simulink model "PlatoonWithLateralControlExample"  (R2021b)
settings: Solver=FixedStepAuto  StartTime=0  StopTime=180  RelTol=1e-3
values from neighbouring files (symbols this model uses):
  C = [1 0 0 0; 0 1 0 0]    [truck_trailer_model.m]
undefined symbols (not defined in the file or in its folder): amp, follow1_pose0, follow2_pose0, follow3_pose0, front_pose0, lead_pose0, Ts, Vx0
libraries: drivingscenarioandsensors x5, sim3dautolib x5, sim3dlib x1
settings Model: PauseTimes=200  Creator=gabep  LastModifiedBy=gabep
settings DataIOCC: SaveFormat=Array  ReturnWorkspaceOutputs=off
settings OptimizationCC: BlockReduction=off  BufferReuse=off
settings DebuggingCC: AlgebraicLoopMsg=none  UnconnectedInputMsg=none  UnconnectedOutputMsg=none  UnconnectedLineMsg=none

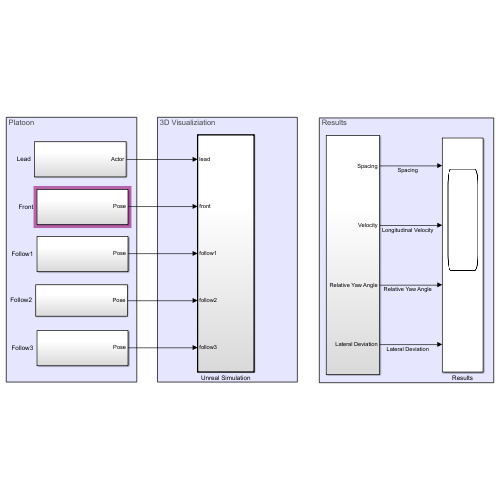
[thumbnail: Simulink's stored preview of the top-level diagram]
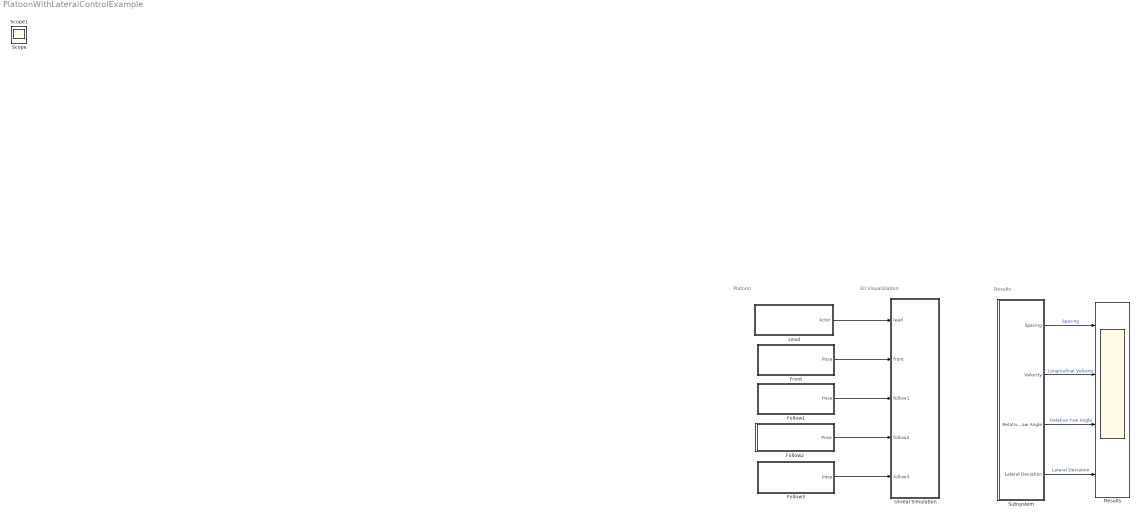
== system PlatoonWithLateralControlExample ==
  note: Results
  note: Platoon
  note: 3D Visualiziation
  Follow1 : Subsystem
      settings: PortSchema="{\"entries\":[{\"content\":{\"sides\":[{\"content\":{\"connectorIds\":[]},\"type\":\"ConnectorPlacement.EquallySpacedRectSide\",\"uuid\":\"e54d76f8-8c49-4840-b6a9-58e08104dcc1\"},{\"content\":{\"connectorIds\":[],\"side\":\"RIGHT\"},\"type\":\"ConnectorPlacement.EquallySpacedRectSide\",\"uuid\":\"16d97aed-590d-4da6-9d09-35159b7cd9d4\"},{\"content\":{\"connectorIds\":[\"Out1\"],\"side\":\"TOP\"},\"type\":\"ConnectorPlacement.EquallySpacedRectSide\",\"uuid\":\"c2bfedc8-00ba-418d-b164-6614631c3f94\"}]},\"type\":\"ConnectorPlacement.EquallySpacedConnector\",\"uuid\":\"51c3c2ba-a1bc-4371-a1ec-9944d72910ba\"}],\"packageUris\":[\"http://schema.mathworks.com/mf0/Connector/R2020b\"],\"version\":\"1.0\"}"
  Follow2 : Subsystem
      settings: PortSchema="{\"entries\":[{\"content\":{\"sides\":[{\"content\":{\"connectorIds\":[]},\"type\":\"ConnectorPlacement.EquallySpacedRectSide\",\"uuid\":\"06893071-ec21-4ffc-a054-06bfa92a0eac\"},{\"content\":{\"connectorIds\":[],\"side\":\"RIGHT\"},\"type\":\"ConnectorPlacement.EquallySpacedRectSide\",\"uuid\":\"1cbc90e1-f519-4952-8f8a-3c170042a637\"},{\"content\":{\"connectorIds\":[\"Out1\"],\"side\":\"TOP\"},\"type\":\"ConnectorPlacement.EquallySpacedRectSide\",\"uuid\":\"b6adb661-09de-4d57-bc58-bfba7e0f462d\"}]},\"type\":\"ConnectorPlacement.EquallySpacedConnector\",\"uuid\":\"b02e6905-9b80-44f2-a3ff-3310e2960530\"}],\"packageUris\":[\"http://schema.mathworks.com/mf0/Connector/R2020b\"],\"version\":\"1.0\"}"
  Follow3 : Subsystem
      settings: PortSchema="{\"entries\":[{\"content\":{\"sides\":[{\"content\":{\"connectorIds\":[]},\"type\":\"ConnectorPlacement.EquallySpacedRectSide\",\"uuid\":\"e54d76f8-8c49-4840-b6a9-58e08104dcc1\"},{\"content\":{\"connectorIds\":[],\"side\":\"RIGHT\"},\"type\":\"ConnectorPlacement.EquallySpacedRectSide\",\"uuid\":\"16d97aed-590d-4da6-9d09-35159b7cd9d4\"},{\"content\":{\"connectorIds\":[\"Out1\"],\"side\":\"TOP\"},\"type\":\"ConnectorPlacement.EquallySpacedRectSide\",\"uuid\":\"c2bfedc8-00ba-418d-b164-6614631c3f94\"}]},\"type\":\"ConnectorPlacement.EquallySpacedConnector\",\"uuid\":\"51c3c2ba-a1bc-4371-a1ec-9944d72910ba\"}],\"packageUris\":[\"http://schema.mathworks.com/mf0/Connector/R2020b\"],\"version\":\"1.0\"}"
  Front : Subsystem
      settings: PortSchema="{\"entries\":[{\"content\":{\"sides\":[{\"content\":{\"connectorIds\":[]},\"type\":\"ConnectorPlacement.EquallySpacedRectSide\",\"uuid\":\"e54d76f8-8c49-4840-b6a9-58e08104dcc1\"},{\"content\":{\"connectorIds\":[],\"side\":\"RIGHT\"},\"type\":\"ConnectorPlacement.EquallySpacedRectSide\",\"uuid\":\"16d97aed-590d-4da6-9d09-35159b7cd9d4\"},{\"content\":{\"connectorIds\":[\"Out1\"],\"side\":\"TOP\"},\"type\":\"ConnectorPlacement.EquallySpacedRectSide\",\"uuid\":\"c2bfedc8-00ba-418d-b164-6614631c3f94\"}]},\"type\":\"ConnectorPlacement.EquallySpacedConnector\",\"uuid\":\"51c3c2ba-a1bc-4371-a1ec-9944d72910ba\"}],\"packageUris\":[\"http://schema.mathworks.com/mf0/Connector/R2020b\"],\"version\":\"1.0\"}"
  Lead : Subsystem
      settings: PortSchema="{\"entries\":[{\"content\":{\"sides\":[{\"content\":{\"connectorIds\":[]},\"type\":\"ConnectorPlacement.EquallySpacedRectSide\",\"uuid\":\"e54d76f8-8c49-4840-b6a9-58e08104dcc1\"},{\"content\":{\"connectorIds\":[],\"side\":\"RIGHT\"},\"type\":\"ConnectorPlacement.EquallySpacedRectSide\",\"uuid\":\"16d97aed-590d-4da6-9d09-35159b7cd9d4\"},{\"content\":{\"connectorIds\":[\"Out1\"],\"side\":\"TOP\"},\"type\":\"ConnectorPlacement.EquallySpacedRectSide\",\"uuid\":\"c2bfedc8-00ba-418d-b164-6614631c3f94\"}]},\"type\":\"ConnectorPlacement.EquallySpacedConnector\",\"uuid\":\"51c3c2ba-a1bc-4371-a1ec-9944d72910ba\"}],\"packageUris\":[\"http://schema.mathworks.com/mf0/Connector/R2020b\"],\"version\":\"1.0\"}"
  Results : Scope  NumInputPorts=4
  Subsystem : Subsystem
  Unreal Simulation : Subsystem  TreatAsAtomicUnit=on
  Scope : Scope
  Scope1 : Scope
  wires:
  Lead/1(Actor) -> Unreal Simulation/1(lead)
  Front/1(Pose) -> Unreal Simulation/2(front)
  Follow1/1(Pose) -> Unreal Simulation/3(follow1)
  Follow2/1(Pose) -> Unreal Simulation/4(follow2)
  Follow3/1(Pose) -> Unreal Simulation/5(follow3)
  Subsystem/1(Spacing) -> Results/1  "Spacing"
  Subsystem/2(Velocity) -> Results/2  "Longitudinal Velocity"
  Subsystem/4(Lateral Deviation) -> Results/4  "Lateral Deviation"
  Subsystem/3(Relative Yaw Angle) -> Results/3  "Relative Yaw Angle"

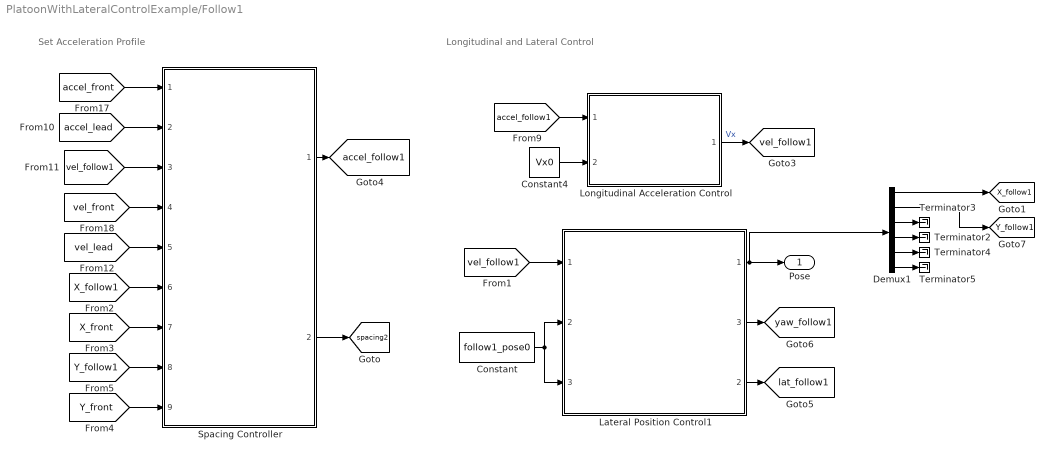
== system PlatoonWithLateralControlExample/Follow1 ==
  note: Set Acceleration Profile
  note: Longitudinal and Lateral Control
  Constant : Constant  Value=follow1_pose0
  Constant4 : Constant  Value=Vx0
  Demux1 : Demux  Outputs=6
  Lateral Position Control1 : Subsystem  ReferencedSubsystem=Lateral_Position_Control
      settings: PortSchema="{\"entries\":[{\"content\":{\"sides\":[{\"content\":{\"connectorIds\":[\"In1\",\"In2\",\"In3\"]},\"type\":\"ConnectorPlacement.EquallySpacedRectSide\",\"uuid\":\"be29c3cb-f330-4838-b745-538466c19ec8\"},{\"content\":{\"connectorIds\":[\"Out1\",\"Out3\",\"Out2\"],\"side\":\"RIGHT\"},\"type\":\"ConnectorPlacement.EquallySpacedRectSide\",\"uuid\":\"f85912df-f35d-4388-8854-cabd9b7a9775\"},{\"content\":{\"connectorIds\":[],\"side\":\"TOP\"},\"type\":\"ConnectorPlacement.EquallySpacedRectSide\",\"uuid\":\"58ed6a5b-2636-4a09-8dd1-9e23de881849\"}]},\"type\":\"ConnectorPlacement.EquallySpacedConnector\",\"uuid\":\"159292d7-4540-43fd-9ff3-bfddba653fcb\"}],\"packageUris\":[\"http://schema.mathworks.com/mf0/Connector/R2020b\"],\"version\":\"1.0\"}"
  Longitudinal Acceleration Control : Subsystem  ReferencedSubsystem=Longitudinal_Acceleration_Control
  Spacing Controller : Subsystem  ReferencedSubsystem=spacing_controller
  Terminator{2..5} (4 alike) : Terminator
  Pose : Outport
  tag scope: X_follow1=global, Y_follow1=global, accel_follow1=global, lat_follow1=global, spacing2=global, vel_follow1=global, yaw_follow1=global
  wires:
  Constant4/1 -> Longitudinal Acceleration Control/2
  [accel_follow1] -> Longitudinal Acceleration Control/1
  Longitudinal Acceleration Control/1 -> [vel_follow1]  "Vx"
  Lateral Position Control1/3 -> [yaw_follow1]
  Lateral Position Control1/2 -> [lat_follow1]
  [vel_follow1] -> Lateral Position Control1/1
  Constant/1 -> Lateral Position Control1/3, Lateral Position Control1/2
  Spacing Controller/2 -> [spacing2]
  [accel_front] -> Spacing Controller/1
  [accel_lead] -> Spacing Controller/2
  [vel_follow1] -> Spacing Controller/3
  [vel_front] -> Spacing Controller/4
  [vel_lead] -> Spacing Controller/5
  Spacing Controller/1 -> [accel_follow1]
  [X_front] -> Spacing Controller/7
  [X_follow1] -> Spacing Controller/6
  Demux1/4 -> Terminator2/1
  Demux1/6 -> Terminator5/1
  Demux1/2 -> [Y_follow1]
  Demux1/1 -> [X_follow1]
  Demux1/5 -> Terminator4/1
  Demux1/3 -> Terminator3/1
  Lateral Position Control1/1 -> Demux1/1, Pose/1
  [Y_front] -> Spacing Controller/9
  [Y_follow1] -> Spacing Controller/8

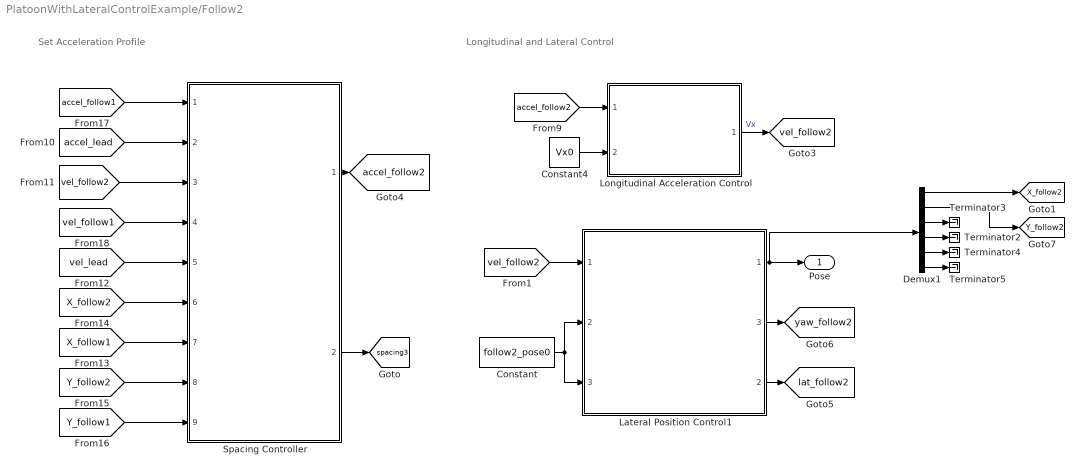
== system PlatoonWithLateralControlExample/Follow2 ==
  note: Set Acceleration Profile
  note: Longitudinal and Lateral Control
  Constant : Constant  Value=follow2_pose0
  Constant4 : Constant  Value=Vx0
  Demux1 : Demux  Outputs=6
  Lateral Position Control1 : Subsystem  ReferencedSubsystem=Lateral_Position_Control
      settings: PortSchema="{\"entries\":[{\"content\":{\"sides\":[{\"content\":{\"connectorIds\":[\"In1\",\"In2\",\"In3\"]},\"type\":\"ConnectorPlacement.EquallySpacedRectSide\",\"uuid\":\"be29c3cb-f330-4838-b745-538466c19ec8\"},{\"content\":{\"connectorIds\":[\"Out1\",\"Out3\",\"Out2\"],\"side\":\"RIGHT\"},\"type\":\"ConnectorPlacement.EquallySpacedRectSide\",\"uuid\":\"f85912df-f35d-4388-8854-cabd9b7a9775\"},{\"content\":{\"connectorIds\":[],\"side\":\"TOP\"},\"type\":\"ConnectorPlacement.EquallySpacedRectSide\",\"uuid\":\"58ed6a5b-2636-4a09-8dd1-9e23de881849\"}]},\"type\":\"ConnectorPlacement.EquallySpacedConnector\",\"uuid\":\"159292d7-4540-43fd-9ff3-bfddba653fcb\"}],\"packageUris\":[\"http://schema.mathworks.com/mf0/Connector/R2020b\"],\"version\":\"1.0\"}"
  Longitudinal Acceleration Control : Subsystem  ReferencedSubsystem=Longitudinal_Acceleration_Control
  Spacing Controller : Subsystem  ReferencedSubsystem=spacing_controller
  Terminator{2..5} (4 alike) : Terminator
  Pose : Outport
  tag scope: X_follow2=global, Y_follow2=global, accel_follow2=global, lat_follow2=global, spacing3=global, vel_follow2=global, yaw_follow2=global
  wires:
  Constant4/1 -> Longitudinal Acceleration Control/2
  [accel_follow2] -> Longitudinal Acceleration Control/1
  Longitudinal Acceleration Control/1 -> [vel_follow2]  "Vx"
  [Y_follow2] -> Spacing Controller/8
  [X_follow1] -> Spacing Controller/7
  Spacing Controller/1 -> [accel_follow2]
  [vel_follow2] -> Spacing Controller/3
  [vel_lead] -> Spacing Controller/5
  [accel_lead] -> Spacing Controller/2
  [Y_follow1] -> Spacing Controller/9
  [X_follow2] -> Spacing Controller/6
  [accel_follow1] -> Spacing Controller/1
  [vel_follow1] -> Spacing Controller/4
  Spacing Controller/2 -> [spacing3]
  Lateral Position Control1/3 -> [yaw_follow2]
  Lateral Position Control1/2 -> [lat_follow2]
  [vel_follow2] -> Lateral Position Control1/1
  Constant/1 -> Lateral Position Control1/3, Lateral Position Control1/2
  Demux1/3 -> Terminator3/1
  Demux1/5 -> Terminator4/1
  Demux1/1 -> [X_follow2]
  Demux1/6 -> Terminator5/1
  Demux1/2 -> [Y_follow2]
  Demux1/4 -> Terminator2/1
  Lateral Position Control1/1 -> Demux1/1, Pose/1

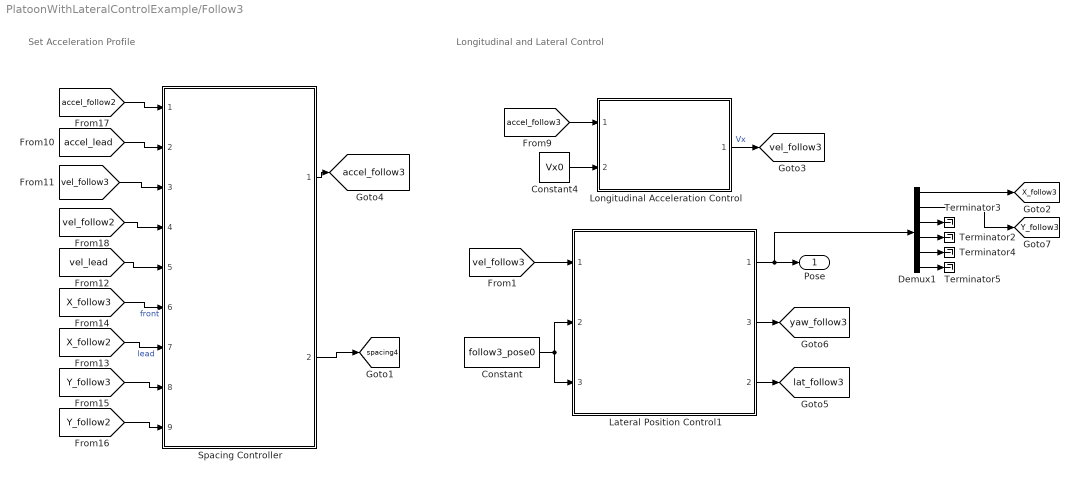
== system PlatoonWithLateralControlExample/Follow3 ==
  note: Set Acceleration Profile
  note: Longitudinal and Lateral Control
  Constant : Constant  Value=follow3_pose0
  Constant4 : Constant  Value=Vx0
  Demux1 : Demux  Outputs=6
  Lateral Position Control1 : Subsystem  ReferencedSubsystem=Lateral_Position_Control
      settings: PortSchema="{\"entries\":[{\"content\":{\"sides\":[{\"content\":{\"connectorIds\":[\"In1\",\"In2\",\"In3\"]},\"type\":\"ConnectorPlacement.EquallySpacedRectSide\",\"uuid\":\"be29c3cb-f330-4838-b745-538466c19ec8\"},{\"content\":{\"connectorIds\":[\"Out1\",\"Out3\",\"Out2\"],\"side\":\"RIGHT\"},\"type\":\"ConnectorPlacement.EquallySpacedRectSide\",\"uuid\":\"f85912df-f35d-4388-8854-cabd9b7a9775\"},{\"content\":{\"connectorIds\":[],\"side\":\"TOP\"},\"type\":\"ConnectorPlacement.EquallySpacedRectSide\",\"uuid\":\"58ed6a5b-2636-4a09-8dd1-9e23de881849\"}]},\"type\":\"ConnectorPlacement.EquallySpacedConnector\",\"uuid\":\"159292d7-4540-43fd-9ff3-bfddba653fcb\"}],\"packageUris\":[\"http://schema.mathworks.com/mf0/Connector/R2020b\"],\"version\":\"1.0\"}"
  Longitudinal Acceleration Control : Subsystem  ReferencedSubsystem=Longitudinal_Acceleration_Control
  Spacing Controller : Subsystem  ReferencedSubsystem=spacing_controller
  Terminator{2..5} (4 alike) : Terminator
  Pose : Outport
  tag scope: X_follow3=global, Y_follow3=global, accel_follow3=global, lat_follow3=global, spacing4=global, vel_follow3=global, yaw_follow3=global
  wires:
  Constant4/1 -> Longitudinal Acceleration Control/2
  [accel_follow3] -> Longitudinal Acceleration Control/1
  Longitudinal Acceleration Control/1 -> [vel_follow3]  "Vx"
  [Y_follow3] -> Spacing Controller/8
  [X_follow2] -> Spacing Controller/7  "lead"
  [vel_follow3] -> Spacing Controller/3
  [vel_lead] -> Spacing Controller/5
  [accel_lead] -> Spacing Controller/2
  [Y_follow2] -> Spacing Controller/9
  [X_follow3] -> Spacing Controller/6  "front"
  [accel_follow2] -> Spacing Controller/1
  [vel_follow2] -> Spacing Controller/4
  Spacing Controller/1 -> [accel_follow3]
  Spacing Controller/2 -> [spacing4]
  Lateral Position Control1/3 -> [yaw_follow3]
  Lateral Position Control1/2 -> [lat_follow3]
  [vel_follow3] -> Lateral Position Control1/1
  Constant/1 -> Lateral Position Control1/3, Lateral Position Control1/2
  Demux1/3 -> Terminator3/1
  Demux1/5 -> Terminator4/1
  Demux1/1 -> [X_follow3]
  Demux1/6 -> Terminator5/1
  Demux1/2 -> [Y_follow3]
  Demux1/4 -> Terminator2/1
  Lateral Position Control1/1 -> Demux1/1, Pose/1

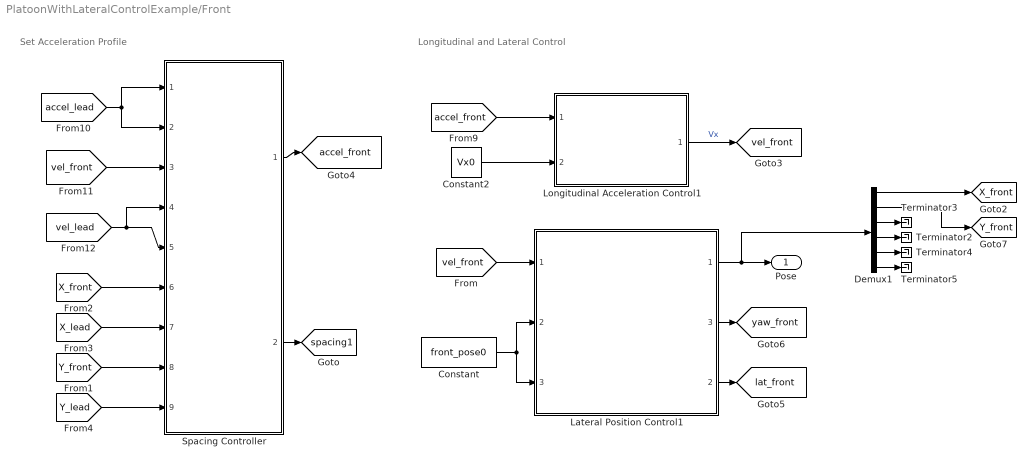
== system PlatoonWithLateralControlExample/Front ==
  note: Longitudinal and Lateral Control
  note: Set Acceleration Profile
  Constant : Constant  Value=front_pose0
  Constant2 : Constant  Value=Vx0
  Demux1 : Demux  Outputs=6
  Lateral Position Control1 : Subsystem  ReferencedSubsystem=Lateral_Position_Control
      settings: PortSchema="{\"entries\":[{\"content\":{\"sides\":[{\"content\":{\"connectorIds\":[\"In1\",\"In2\",\"In3\"]},\"type\":\"ConnectorPlacement.EquallySpacedRectSide\",\"uuid\":\"be29c3cb-f330-4838-b745-538466c19ec8\"},{\"content\":{\"connectorIds\":[\"Out1\",\"Out3\",\"Out2\"],\"side\":\"RIGHT\"},\"type\":\"ConnectorPlacement.EquallySpacedRectSide\",\"uuid\":\"f85912df-f35d-4388-8854-cabd9b7a9775\"},{\"content\":{\"connectorIds\":[],\"side\":\"TOP\"},\"type\":\"ConnectorPlacement.EquallySpacedRectSide\",\"uuid\":\"58ed6a5b-2636-4a09-8dd1-9e23de881849\"}]},\"type\":\"ConnectorPlacement.EquallySpacedConnector\",\"uuid\":\"159292d7-4540-43fd-9ff3-bfddba653fcb\"}],\"packageUris\":[\"http://schema.mathworks.com/mf0/Connector/R2020b\"],\"version\":\"1.0\"}"
  Longitudinal Acceleration Control1 : Subsystem  ReferencedSubsystem=Longitudinal_Acceleration_Control
  Spacing Controller : Subsystem  ReferencedSubsystem=spacing_controller
  Terminator{2..5} (4 alike) : Terminator
  Pose : Outport
  tag scope: X_front=global, Y_front=global, accel_front=global, lat_front=global, spacing1=global, vel_front=global, yaw_front=global
  wires:
  [accel_lead] -> Spacing Controller/2, Spacing Controller/1
  [vel_front] -> Spacing Controller/3
  [vel_lead] -> Spacing Controller/5, Spacing Controller/4
  Spacing Controller/1 -> [accel_front]
  Constant/1 -> Lateral Position Control1/3, Lateral Position Control1/2
  Constant2/1 -> Longitudinal Acceleration Control1/2
  [accel_front] -> Longitudinal Acceleration Control1/1
  Lateral Position Control1/2 -> [lat_front]
  Longitudinal Acceleration Control1/1 -> [vel_front]  "Vx"
  Lateral Position Control1/3 -> [yaw_front]
  [vel_front] -> Lateral Position Control1/1
  [X_front] -> Spacing Controller/6
  [X_lead] -> Spacing Controller/7
  Spacing Controller/2 -> [spacing1]
  Demux1/4 -> Terminator2/1
  Demux1/6 -> Terminator5/1
  Demux1/2 -> [Y_front]
  Demux1/1 -> [X_front]
  Demux1/5 -> Terminator4/1
  Demux1/3 -> Terminator3/1
  Lateral Position Control1/1 -> Pose/1, Demux1/1
  [Y_lead] -> Spacing Controller/9
  [Y_front] -> Spacing Controller/8

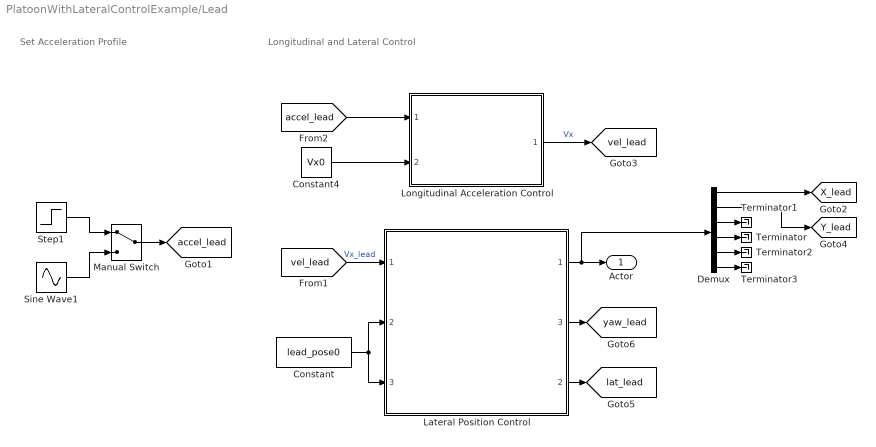
== system PlatoonWithLateralControlExample/Lead ==
  note: Set Acceleration Profile
  note: Longitudinal and Lateral Control
  Constant : Constant  Value=lead_pose0
  Constant4 : Constant  Value=Vx0
  Demux : Demux  Outputs=6
  Lateral Position Control : Subsystem  ReferencedSubsystem=Lateral_Position_Control
      settings: PortSchema="{\"entries\":[{\"content\":{\"sides\":[{\"content\":{\"connectorIds\":[\"In1\",\"In2\",\"In3\"]},\"type\":\"ConnectorPlacement.EquallySpacedRectSide\",\"uuid\":\"be29c3cb-f330-4838-b745-538466c19ec8\"},{\"content\":{\"connectorIds\":[\"Out1\",\"Out3\",\"Out2\"],\"side\":\"RIGHT\"},\"type\":\"ConnectorPlacement.EquallySpacedRectSide\",\"uuid\":\"f85912df-f35d-4388-8854-cabd9b7a9775\"},{\"content\":{\"connectorIds\":[],\"side\":\"TOP\"},\"type\":\"ConnectorPlacement.EquallySpacedRectSide\",\"uuid\":\"58ed6a5b-2636-4a09-8dd1-9e23de881849\"}]},\"type\":\"ConnectorPlacement.EquallySpacedConnector\",\"uuid\":\"159292d7-4540-43fd-9ff3-bfddba653fcb\"}],\"packageUris\":[\"http://schema.mathworks.com/mf0/Connector/R2020b\"],\"version\":\"1.0\"}"
  Longitudinal Acceleration Control : Subsystem  ReferencedSubsystem=Longitudinal_Acceleration_Control
  Manual Switch : ManualSwitch
  Sine Wave1 : Sin  Amplitude=amp  SampleTime=0
  Step1 : Step  Time=0  After=0  SampleTime=0
  Terminator{,1..3} (4 alike) : Terminator
  Actor : Outport
  tag scope: X_lead=global, Y_lead=global, accel_lead=global, lat_lead=global, vel_lead=global, yaw_lead=global
  wires:
  Constant4/1 -> Longitudinal Acceleration Control/2
  Longitudinal Acceleration Control/1 -> [vel_lead]  "Vx"
  [accel_lead] -> Longitudinal Acceleration Control/1
  Step1/1 -> Manual Switch/1
  Manual Switch/1 -> [accel_lead]
  Sine Wave1/1 -> Manual Switch/2
  Lateral Position Control/3 -> [yaw_lead]
  Lateral Position Control/2 -> [lat_lead]
  Constant/1 -> Lateral Position Control/2, Lateral Position Control/3
  [vel_lead] -> Lateral Position Control/1  "Vx_lead"
  Demux/2 -> [Y_lead]
  Lateral Position Control/1 -> Demux/1, Actor/1
  Demux/3 -> Terminator1/1
  Demux/1 -> [X_lead]
  Demux/4 -> Terminator/1
  Demux/5 -> Terminator2/1
  Demux/6 -> Terminator3/1

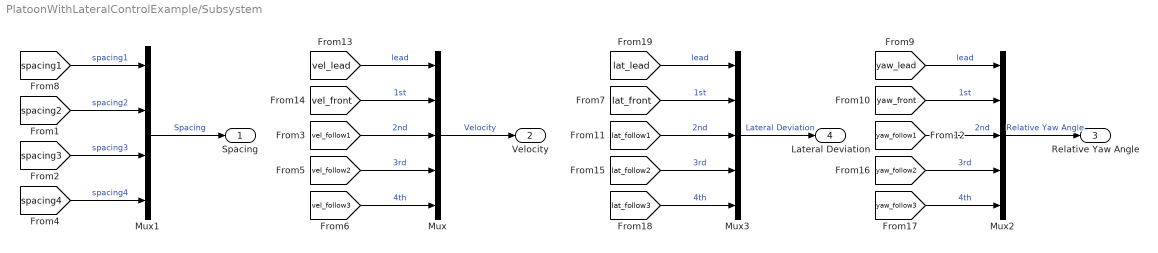
== system PlatoonWithLateralControlExample/Subsystem ==
  Mux : Mux  Inputs=5
  Mux1 : Mux
  Mux2 : Mux  Inputs=5
  Mux3 : Mux  Inputs=5
  Spacing : Outport
  Velocity : Outport  Port=2
  Relative Yaw Angle : Outport  Port=3
  Lateral Deviation : Outport  Port=4
  wires:
  [vel_follow2] -> Mux/4  "3rd"
  [vel_lead] -> Mux/1  "lead"
  [vel_front] -> Mux/2  "1st"
  [spacing3] -> Mux1/3  "spacing3"
  [vel_follow1] -> Mux/3  "2nd"
  [spacing1] -> Mux1/1  "spacing1"
  [spacing4] -> Mux1/4  "spacing4"
  [vel_follow3] -> Mux/5  "4th"
  [spacing2] -> Mux1/2  "spacing2"
  Mux/1 -> Velocity/1  "Velocity"
  Mux1/1 -> Spacing/1  "Spacing"
  Mux2/1 -> Relative Yaw Angle/1  "Relative Yaw Angle"
  [yaw_follow3] -> Mux2/5  "4th"
  [yaw_follow1] -> Mux2/3  "2nd"
  [yaw_front] -> Mux2/2  "1st"
  [yaw_follow2] -> Mux2/4  "3rd"
  [yaw_lead] -> Mux2/1  "lead"
  [lat_lead] -> Mux3/1  "lead"
  [lat_follow1] -> Mux3/3  "2nd"
  [lat_follow2] -> Mux3/4  "3rd"
  Mux3/1 -> Lateral Deviation/1  "Lateral Deviation"
  [lat_follow3] -> Mux3/5  "4th"
  [lat_front] -> Mux3/2  "1st"

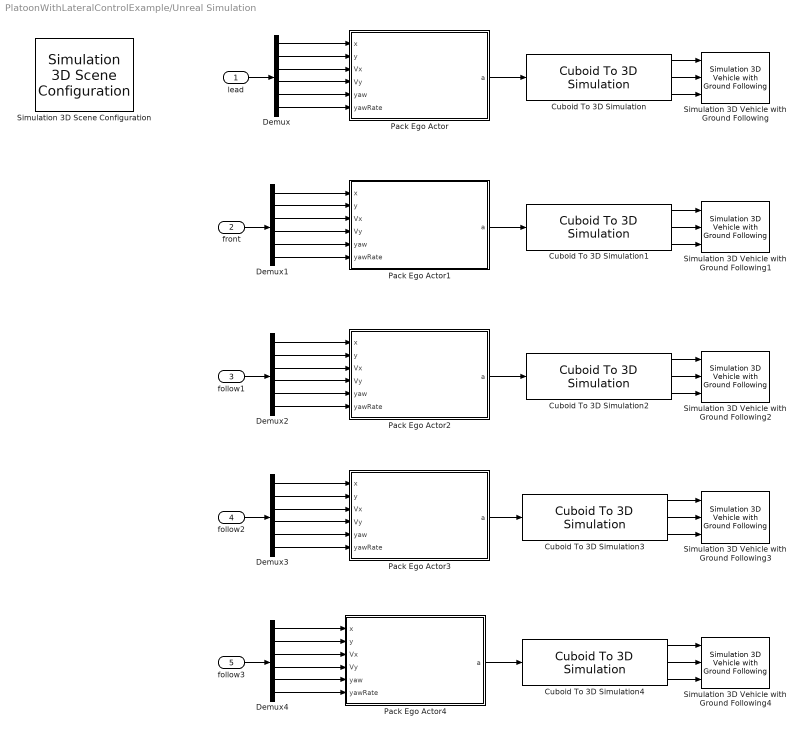
== system PlatoonWithLateralControlExample/Unreal Simulation ==
  lead : Inport
  front : Inport  Port=2
  follow1 : Inport  Port=3
  follow2 : Inport  Port=4
  follow3 : Inport  Port=5
  Cuboid To 3D Simulation{,1..4} (5 alike) : drivingscenarioandsensors/Cuboid To 3D Simulation  SpecifyActorID=off  ActorIDToConvert=1  SimulateUsing=Interpreted execution
      settings: SourceProductBaseCode=DR
  Demux{,1..4} (5 alike) : Demux  Outputs=6
  Pack Ego Actor : MATLAB Function  TreatAsAtomicUnit=on  mask{egoActorID=1}
      mask prompts: egoActorID "Ego Actor ID"
  Pack Ego Actor1 : MATLAB Function  TreatAsAtomicUnit=on  mask{egoActorID=1}
      mask prompts: egoActorID "Ego Actor ID"
  Pack Ego Actor2 : MATLAB Function  TreatAsAtomicUnit=on  mask{egoActorID=1}
      mask prompts: egoActorID "Ego Actor ID"
  Pack Ego Actor3 : MATLAB Function  TreatAsAtomicUnit=on  mask{egoActorID=1}
      mask prompts: egoActorID "Ego Actor ID"
  Pack Ego Actor4 : MATLAB Function  TreatAsAtomicUnit=on  mask{egoActorID=1}
      mask prompts: egoActorID "Ego Actor ID"
  Simulation 3D Scene Configuration : sim3dlib/Simulation 3D Scene Configuration  Priority=0  ProjectFormat_internal=Unreal Executable  ProjectFormat=Unreal Executable  SceneDesc=Curved road  ProjectName=C:\ProgramData\MATLAB\SupportPackages\R2021b\toolbox\shared\sim3dprojects\driving\RoadRunnerScenes\WindowsPackage\RRScene.exe  ScenePath=/Game/Maps/RRHighway  vehTagList={'Scene Origin';'SimulinkVehicle1';'SimulinkVehicle2';'SimulinkVehicle3';'SimulinkVehicle4';'SimulinkVehicle5'}  vehTag=SimulinkVehicle5  OpVisEn=off  Ts=Ts  EnableWindow=on  EnableWeather=off  SunAltitude=-43.200  SunAzimuth=54.0  clouds=7.0  wind=2.0  fog=0  rain=0  sensorTag=MainCamera1  sensorId=1  sensorName=MainCamera1  mountLoc=Origin  offsetFlag=off  tmountOffset=[0, 0, 0]  rmountOffset=[0, 0, 0]  HorizontalResolution=1280  VerticalResolution=720  HorizontalFOV=60  mountPoint=[0 0 0]  mountOrientation=[0 0 0]  aMode=3  ID=1
      settings: SourceProductBaseCode=AE,DR,UV,VE
      settings: AttributesFormatString=|
      | -------------------------------------
      | SceneName = %<SceneDesc>
      | Priority = %<Priority>
  Simulation 3D Vehicle with Ground Following : sim3dautolib/Simulation 3D Vehicle with Ground Following  Priority=-1  PassVehMesh=Box truck  PassVehMesh_Internal=Box truck  MeshPath=/MathWorksSimulation/Vehicles/Muscle/Meshes/SK_MuscleCar.SK_MuscleCar  TrackWidth=1.9  WheelBase=3  WheelRadius=0.35  VehColor=Blue  VehColor_Internal=Blue  InitialPos=[0,0,0]  InitialRot=[0, 0, 0]  ActorName=SimulinkVehicle1  SampleTime=-1  ActorType=SimulinkVehicle  ID=1  aMode=3  ActorTag=SimulinkVehicle1  CoordinateScheme=ISO  VehLightsControl=off  HeadlightColor=[ 1, 1, 1 ]  HighBeamIntensity=100000  LowBeamIntensity=60000  HighBeamConeAngle=70  LowBeamConeAngle=70  LeftHeadlightOrientation=[ 0, 0 ]  RightHeadlightOrientation=[ 0, 0 ]  BrakelightIntensity=500  ReverselightIntensity=500  SignallightIntensity=500  SignallightPeriod=1  SignalPulseWidth=50  TransformOutportEnabled=off
      settings: SourceProductBaseCode=AE,DR,UV,VE
  Simulation 3D Vehicle with Ground Following1 : sim3dautolib/Simulation 3D Vehicle with Ground Following  Priority=-1  PassVehMesh=Box truck  PassVehMesh_Internal=Box truck  MeshPath=/MathWorksSimulation/Vehicles/Muscle/Meshes/SK_MuscleCar.SK_MuscleCar  TrackWidth=1.9  WheelBase=3  WheelRadius=0.35  VehColor=Orange  VehColor_Internal=Orange  InitialPos=[0, 0, 0]  InitialRot=[0, 0, 0]  ActorName=SimulinkVehicle2  SampleTime=-1  ActorType=SimulinkVehicle  ID=2  aMode=3  ActorTag=SimulinkVehicle2  CoordinateScheme=ISO  VehLightsControl=off  HeadlightColor=[ 1, 1, 1 ]  HighBeamIntensity=100000  LowBeamIntensity=60000  HighBeamConeAngle=70  LowBeamConeAngle=70  LeftHeadlightOrientation=[ 0, 0 ]  RightHeadlightOrientation=[ 0, 0 ]  BrakelightIntensity=500  ReverselightIntensity=500  SignallightIntensity=500  SignallightPeriod=1  SignalPulseWidth=50  TransformOutportEnabled=off
      settings: SourceProductBaseCode=AE,DR,UV,VE
  Simulation 3D Vehicle with Ground Following2 : sim3dautolib/Simulation 3D Vehicle with Ground Following  Priority=-1  PassVehMesh=Box truck  PassVehMesh_Internal=Box truck  MeshPath=/MathWorksSimulation/Vehicles/Muscle/Meshes/SK_MuscleCar.SK_MuscleCar  TrackWidth=1.9  WheelBase=3  WheelRadius=0.35  VehColor=Yellow  VehColor_Internal=Yellow  InitialPos=[0, 0, 0]  InitialRot=[0, 0, 0]  ActorName=SimulinkVehicle3  SampleTime=-1  ActorType=SimulinkVehicle  ID=3  aMode=3  ActorTag=SimulinkVehicle3  CoordinateScheme=ISO  VehLightsControl=off  HeadlightColor=[ 1, 1, 1 ]  HighBeamIntensity=100000  LowBeamIntensity=60000  HighBeamConeAngle=70  LowBeamConeAngle=70  LeftHeadlightOrientation=[ 0, 0 ]  RightHeadlightOrientation=[ 0, 0 ]  BrakelightIntensity=500  ReverselightIntensity=500  SignallightIntensity=500  SignallightPeriod=1  SignalPulseWidth=50  TransformOutportEnabled=off
      settings: SourceProductBaseCode=AE,DR,UV,VE
  Simulation 3D Vehicle with Ground Following3 : sim3dautolib/Simulation 3D Vehicle with Ground Following  Priority=-1  PassVehMesh=Box truck  PassVehMesh_Internal=Box truck  MeshPath=/MathWorksSimulation/Vehicles/Muscle/Meshes/SK_MuscleCar.SK_MuscleCar  TrackWidth=1.9  WheelBase=3  WheelRadius=0.35  VehColor=White  VehColor_Internal=White  InitialPos=[0, 0, 0]  InitialRot=[0, 0, 0]  ActorName=SimulinkVehicle4  SampleTime=-1  ActorType=SimulinkVehicle  ID=4  aMode=3  ActorTag=SimulinkVehicle4  CoordinateScheme=ISO  VehLightsControl=off  HeadlightColor=[ 1, 1, 1 ]  HighBeamIntensity=100000  LowBeamIntensity=60000  HighBeamConeAngle=70  LowBeamConeAngle=70  LeftHeadlightOrientation=[ 0, 0 ]  RightHeadlightOrientation=[ 0, 0 ]  BrakelightIntensity=500  ReverselightIntensity=500  SignallightIntensity=500  SignallightPeriod=1  SignalPulseWidth=50  TransformOutportEnabled=off
      settings: SourceProductBaseCode=AE,DR,UV,VE
  Simulation 3D Vehicle with Ground Following4 : sim3dautolib/Simulation 3D Vehicle with Ground Following  Priority=-1  PassVehMesh=Box truck  PassVehMesh_Internal=Box truck  MeshPath=/MathWorksSimulation/Vehicles/Muscle/Meshes/SK_MuscleCar.SK_MuscleCar  TrackWidth=1.9  WheelBase=3  WheelRadius=0.35  VehColor=Silver  VehColor_Internal=Silver  InitialPos=[0, 0, 0]  InitialRot=[0, 0, 0]  ActorName=SimulinkVehicle5  SampleTime=-1  ActorType=SimulinkVehicle  ID=5  aMode=3  ActorTag=SimulinkVehicle5  CoordinateScheme=ISO  VehLightsControl=off  HeadlightColor=[ 1, 1, 1 ]  HighBeamIntensity=100000  LowBeamIntensity=60000  HighBeamConeAngle=70  LowBeamConeAngle=70  LeftHeadlightOrientation=[ 0, 0 ]  RightHeadlightOrientation=[ 0, 0 ]  BrakelightIntensity=500  ReverselightIntensity=500  SignallightIntensity=500  SignallightPeriod=1  SignalPulseWidth=50  TransformOutportEnabled=off
      settings: SourceProductBaseCode=AE,DR,UV,VE
  wires:
  Demux/4 -> Pack Ego Actor/4(Vy)
  Demux/6 -> Pack Ego Actor/6(yawRate)
  Demux/1 -> Pack Ego Actor/1(x)
  Demux/5 -> Pack Ego Actor/5(yaw)
  Demux/3 -> Pack Ego Actor/3(Vx)
  Pack Ego Actor/1(a) -> Cuboid To 3D Simulation/1
  lead/1 -> Demux/1
  Demux1/3 -> Pack Ego Actor1/3(Vx)
  Demux1/5 -> Pack Ego Actor1/5(yaw)
  Demux1/1 -> Pack Ego Actor1/1(x)
  Demux1/4 -> Pack Ego Actor1/4(Vy)
  Demux1/6 -> Pack Ego Actor1/6(yawRate)
  front/1 -> Demux1/1
  Demux2/6 -> Pack Ego Actor2/6(yawRate)
  Demux2/1 -> Pack Ego Actor2/1(x)
  Demux2/5 -> Pack Ego Actor2/5(yaw)
  Demux2/2 -> Pack Ego Actor2/2(y)
  Demux2/3 -> Pack Ego Actor2/3(Vx)
  Demux2/4 -> Pack Ego Actor2/4(Vy)
  Demux3/6 -> Pack Ego Actor3/6(yawRate)
  Demux3/1 -> Pack Ego Actor3/1(x)
  Demux3/5 -> Pack Ego Actor3/5(yaw)
  Demux3/2 -> Pack Ego Actor3/2(y)
  Demux3/3 -> Pack Ego Actor3/3(Vx)
  Demux3/4 -> Pack Ego Actor3/4(Vy)
  Demux4/6 -> Pack Ego Actor4/6(yawRate)
  Demux4/1 -> Pack Ego Actor4/1(x)
  Demux4/5 -> Pack Ego Actor4/5(yaw)
  Demux4/2 -> Pack Ego Actor4/2(y)
  Demux4/3 -> Pack Ego Actor4/3(Vx)
  Demux4/4 -> Pack Ego Actor4/4(Vy)
  follow3/1 -> Demux4/1
  Pack Ego Actor4/1(a) -> Cuboid To 3D Simulation4/1
  follow2/1 -> Demux3/1
  Pack Ego Actor3/1(a) -> Cuboid To 3D Simulation3/1
  Pack Ego Actor2/1(a) -> Cuboid To 3D Simulation2/1
  follow1/1 -> Demux2/1
  Demux/2 -> Pack Ego Actor/2(y)
  Demux1/2 -> Pack Ego Actor1/2(y)
  Cuboid To 3D Simulation1/3 -> Simulation 3D Vehicle with Ground Following1/3
  Cuboid To 3D Simulation2/3 -> Simulation 3D Vehicle with Ground Following2/3
  Cuboid To 3D Simulation/3 -> Simulation 3D Vehicle with Ground Following/3
  Cuboid To 3D Simulation3/2 -> Simulation 3D Vehicle with Ground Following3/2
  Cuboid To 3D Simulation4/2 -> Simulation 3D Vehicle with Ground Following4/2
  Cuboid To 3D Simulation1/2 -> Simulation 3D Vehicle with Ground Following1/2
  Cuboid To 3D Simulation4/1 -> Simulation 3D Vehicle with Ground Following4/1
  Cuboid To 3D Simulation2/2 -> Simulation 3D Vehicle with Ground Following2/2
  Cuboid To 3D Simulation3/3 -> Simulation 3D Vehicle with Ground Following3/3
  Cuboid To 3D Simulation1/1 -> Simulation 3D Vehicle with Ground Following1/1
  Cuboid To 3D Simulation/2 -> Simulation 3D Vehicle with Ground Following/2
  Cuboid To 3D Simulation/1 -> Simulation 3D Vehicle with Ground Following/1
  Cuboid To 3D Simulation3/1 -> Simulation 3D Vehicle with Ground Following3/1
  Cuboid To 3D Simulation2/1 -> Simulation 3D Vehicle with Ground Following2/1
  Pack Ego Actor1/1(a) -> Cuboid To 3D Simulation1/1
  Cuboid To 3D Simulation4/3 -> Simulation 3D Vehicle with Ground Following4/3

== matlab function PlatoonWithLateralControlExample/Unreal Simulation/Pack Ego Actor1 ==
  data: x input; a output Bus: BusVehiclePose size=1; y input; Vx input; Vy input; yaw input; yawRate input
function a = packEgo(x,y,Vx,Vy,yaw,yawRate)
% Pack ego information into a single ego actor bus
%
% Important note:
% Output is a bus of type BusVehiclePose. This bus must match the bus 
% elements expected by Scenario Reader. You can view the 
% bus association using 'Edit Data' in the menu above.

a = struct(...
    'ActorID', 1,...
    'Position', [x y 0], ...
    'Velocity', [Vx Vy 0], ...
    'Roll', 0, ...
    'Pitch', 0, ...
    'Yaw', yaw, ...
    'AngularVelocity', [0 0 yawRate]);

== matlab function PlatoonWithLateralControlExample/Unreal Simulation/Pack Ego Actor2 ==
  data: x input; a output Bus: BusVehiclePose size=1; y input; Vx input; Vy input; yaw input; yawRate input
function a = packEgo(x,y,Vx,Vy,yaw,yawRate)
% Pack ego information into a single ego actor bus
%
% Important note:
% Output is a bus of type BusVehiclePose. This bus must match the bus 
% elements expected by Scenario Reader. You can view the 
% bus association using 'Edit Data' in the menu above.

a = struct(...
    'ActorID', 1,...
    'Position', [x y 0], ...
    'Velocity', [Vx Vy 0], ...
    'Roll', 0, ...
    'Pitch', 0, ...
    'Yaw', yaw, ...
    'AngularVelocity', [0 0 yawRate]);

== matlab function PlatoonWithLateralControlExample/Unreal Simulation/Pack Ego Actor3 ==
  data: x input; a output Bus: BusVehiclePose size=1; y input; Vx input; Vy input; yaw input; yawRate input
function a = packEgo(x,y,Vx,Vy,yaw,yawRate)
% Pack ego information into a single ego actor bus
%
% Important note:
% Output is a bus of type BusVehiclePose. This bus must match the bus 
% elements expected by Scenario Reader. You can view the 
% bus association using 'Edit Data' in the menu above.

a = struct(...
    'ActorID', 1,...
    'Position', [x y 0], ...
    'Velocity', [Vx Vy 0], ...
    'Roll', 0, ...
    'Pitch', 0, ...
    'Yaw', yaw, ...
    'AngularVelocity', [0 0 yawRate]);

== matlab function PlatoonWithLateralControlExample/Unreal Simulation/Pack Ego Actor4 ==
  data: x input; a output Bus: BusVehiclePose size=1; y input; Vx input; Vy input; yaw input; yawRate input
function a = packEgo(x,y,Vx,Vy,yaw,yawRate)
% Pack ego information into a single ego actor bus
%
% Important note:
% Output is a bus of type BusVehiclePose. This bus must match the bus 
% elements expected by Scenario Reader. You can view the 
% bus association using 'Edit Data' in the menu above.

a = struct(...
    'ActorID', 1,...
    'Position', [x y 0], ...
    'Velocity', [Vx Vy 0], ...
    'Roll', 0, ...
    'Pitch', 0, ...
    'Yaw', yaw, ...
    'AngularVelocity', [0 0 yawRate]);

== matlab function PlatoonWithLateralControlExample/Unreal Simulation/Pack Ego Actor ==
  data: x input; a output Bus: BusVehiclePose size=1; y input; Vx input; Vy input; yaw input; yawRate input
function a = packEgo(x,y,Vx,Vy,yaw,yawRate)
% Pack ego information into a single ego actor bus
%
% Important note:
% Output is a bus of type BusVehiclePose. This bus must match the bus 
% elements expected by Scenario Reader. You can view the 
% bus association using 'Edit Data' in the menu above.

a = struct(...
    'ActorID', 1,...
    'Position', [x y 0], ...
    'Velocity', [Vx Vy 0], ...
    'Roll', 0, ...
    'Pitch', 0, ...
    'Yaw', yaw, ...
    'AngularVelocity', [0 0 yawRate]);
